simulink model "Naters"  (R2016a)
settings: Solver=FixedStepAuto  StartTime=1  StopTime=60*24*3  FixedStep=1  RelTol=1e-3
InitFcn:
  | %open the initialization function as a structure s
  | model = bdroot;
  | [t,sample_time,k,Text,Text_ini,Tin_sp,rad_90,step,Qdot_dem, Design,T_primary] = system_init(model);
  | %clear ans
  | 
  | 
  | % time vector
  | %t=s.t;
  | t_step = step;
  | time_u = 1;
  | %sample_time = s.sample_time;
  | 
  | % declare parameters
  | Text_D = Design(1);
  | Tin_D = Design(2);
  | Ts_D = Design(3);
  | Tr_D = Design(4);
  | mdot_d_w = Design(5);
  | Qdot_dem = Qdot_dem;
  | %L_ini= L_ini;
  | 
  | %Text_D = s.Design(1);
  | %Tin_D = s.Design(2);
  | %Ts_D = s.Design(3);
  | %Tr_D = s.Design(4);
  | %mdot_d_w = s.Design(5);
  | %Qdot_dem = s.Qdot_dem;
  | %L_ini= s.L_ini;
  | 
  | %Ab_c = Ab_c;
  | %Bb_c = Bb_c;
  | %Tin_sp = Tin_sp.signals.values;
  | Text = Text.signals.values;
  | Rad_90 = rad_90.signals.values;
  | 
  | % k parameters for heat pump model
  | K = k;
values from neighbouring files (symbols this model uses):
  Design = [Text_D, Tin_D, Ts_D, Tr_D, mdot_d_w]    [get_param_building.m]
  k = K    [Frontend.m]    (also in tetsts.m = 2)
  rad_90 = struct('time', t, 'signals', struct('values', rad_90_data(1:length(t))))    [Frontend.m]    (also in system_init.m = kron(rad_90,ones(60,1)); tetsts.m = rad_90(time))
  sample_time = 60    [Frontend.m]    (also in system_init.m = 1; tetsts.m = [1 60 300 900])
  T_primary = 10    [Frontend.m]
undefined symbols (not defined in the file or in its folder): DiscIntNeverNeededParam
libraries: simulink x25, dspsigops x1, carnot x1
(part 1 of 2)
settings Model: Creator=frederic.amblard  LastModifiedBy=frederic.amblard
settings DataIOCC: ExternalInput=[t, Ab_c, Bb_c, Text, Tin_sp]  FinalStateName=NatersV4_cleanV2xFinal  InitialState=NatersV4_cleanV2xFinal  SaveCompleteFinalSimState=on  SaveFormat=Structure

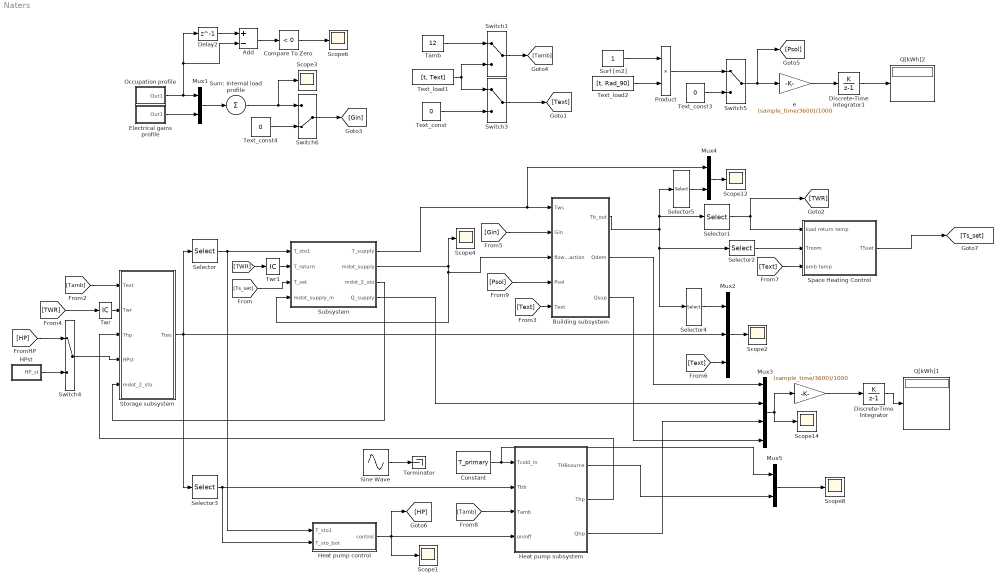
== system Naters ==
  . : Gain  Gain=(sample_time/3600)/1000  SaturateOnIntegerOverflow=on  OutDataTypeStr=Inherit: Same as input  ParamDataTypeStr=Inherit: Same as input
  Add : Sum  Inputs=+-
  Building subsystem : Subsystem
  Compare To Zero : simulink/Logic and Bit Operations/Compare To Zero  relop=<  OutDataTypeStr=uint8
  Constant : Constant  Value=T_primary
  Delay2 : Delay  DelayLength=1  InitialCondition=0
  Discrete-Time Integrator : DiscreteIntegrator  IntegratorMethod=Accumulation: Forward Euler  InitialConditionSetting=State (most efficient)  SampleTime=-1  ICPrevOutput=DiscIntNeverNeededParam  ICPrevScaledInput=DiscIntNeverNeededParam
  Discrete-Time Integrator1 : DiscreteIntegrator  IntegratorMethod=Accumulation: Forward Euler  InitialConditionSetting=State (most efficient)  SampleTime=-1  ICPrevOutput=DiscIntNeverNeededParam  ICPrevScaledInput=DiscIntNeverNeededParam
  Electrical gains profile : Subsystem  mask{period=24*3600/sample_time, rep_seq_t=[0 1 6 7 8 9 11 12 13 18 19 20 22 23]*3600/sample_time, rep_seq_d=[1 5 1 1 1 2 1 1 4 2 1 2 1 1]*3600/sample_time, rep_seq_y=[105 55 392.5 457.5 420 55 250 55 120 170 615 420 442.5 355]*3600/sample_time}
      mask prompts: period "Timeperiod in h"; rep_seq_t "Time values in h"; rep_seq_d "Duration in h"; rep_seq_y "Output values"
  HPst : Subsystem  mask{period=24*3600/sample_time, rep_seq_t=[0 6 7 8 9 11 12 13 14 15 17 18 20 21 22]*3600/sample_time, rep_seq_d=[6 1 1 1 2 1 1 1 1 2 1 2 1 1 2]*3600/sample_time, rep_seq_y=[1 1 1 0 0 0 1 1 1 0 0 1 1 1 1]*3600/sample_time}
      mask prompts: period "Timeperiod in h"; rep_seq_t "Time values in h"; rep_seq_d "Duration in h"; rep_seq_y "Output values"
  Heat pump control : Subsystem
  Heat pump subsystem : Subsystem  mask{K=K, caph=80000, capc=50000, cp=4185, DT=4, UA=7, Qdot_D=Qdot_dem}
      mask prompts: K "Param K"; caph "Thermal capacity hot side [J/K]"; capc "Thermal capacity cold side [J/K]"; cp "Heat capacity of water [J/(kg·K)]"; DT "Delta temperature fixed cold side"; UA "Heat loss coefficient [W/K]"; Qdot_D "Design thermal power [W]"
      mask init:
      | mcdot = 1000*Qdot_D/(DT*cp) / 1000; % mass flow [kg/s]
  Mux1 : Mux  Inputs=2
  Mux2 : Mux  Inputs=3
  Mux3 : Mux
  Mux4 : Mux  Inputs=2
  Mux5 : Mux  Inputs=2
  Occupation profile : Subsystem  mask{period=24*3600/sample_time, rep_seq_t=[0 6 7 8 9 11 12 13 14 15 17 18 20 21 22]*3600/sample_time, rep_seq_d=[6 1 1 1 2 1 1 1 1 2 1 2 1 1 2]*3600/sample_time, rep_seq_y=[4 2 3 2 0 1 3 2 1 0 1 2 4 3 4]*60*3600/sample_time}
      mask prompts: period "Timeperiod in h"; rep_seq_t "Time values in h"; rep_seq_d "Duration in h"; rep_seq_y "Output values"
  Product : Product
  Q[kWh]1 : Display
  Q[kWh]2 : Display
  Scope{1..4,6,8,12,14} (8 alike) : Scope
  Selector : Selector  InputPortWidth=3  IndexOptions=Index vector (dialog)  Indices=[1]  OutputSizes=1
  Selector1 : Selector  InputPortWidth=5  IndexOptions=Index vector (dialog)  Indices=[4]  OutputSizes=1
  Selector2 : Selector  InputPortWidth=5  IndexOptions=Index vector (dialog)  Indices=[5]  OutputSizes=1
  Selector3 : Selector  InputPortWidth=3  IndexOptions=Index vector (dialog)  Indices=[3]  OutputSizes=1
  Selector4 : Selector  InputPortWidth=5  IndexOptions=Index vector (dialog)  Indices=[1, 4, 5]  OutputSizes=1
  Selector5 : Selector  InputPortWidth=5  IndexOptions=Index vector (dialog)  Indices=[1, 2, 3, 4]  OutputSizes=1
  Sine Wave : Sin  SineType=Sample based  Bias=10  Samples=sample_time*100  SampleTime=1  Offset=100
  Space Heating Control : Subsystem  mask{Tset=Tin_D, Tsetn=Tin_D, Q_LOC=Qdot_dem, Td_in=Ts_D, Td_out=Tr_D, Tambd=Text_D, n_rad=1}
      mask prompts: Tset "desired room day Temperature [°C]"; Tsetn "desired room night Temperature [°C]"; Q_LOC "design heat load [W]"; Td_in "design inlet temperature of the heating system [°C]"; Td_out "design outlet temperature of the heating system [°C]"; Tambd "design outdoor temperature"; n_rad "radiatior exponent"
      mask init:
      | dTd = 0.5*(Td_in + Td_out) - Tset;
      | dTdn = 0.5*(Td_in + Td_out) - Tsetn;
  Storage subsystem : Subsystem
  Subsystem : Subsystem
  Sum: Internal load profile : Sum  Inputs=+
  Surf [m2] : Constant
  Switch{1,3..5} (4 alike) : ManualSwitch
  Switch6 : ManualSwitch  CurrentSetting=0
  Tamb : Constant  Value=12
  Terminator : Terminator
  Text_const : Constant  Value=0
  Text_const3 : Constant  Value=0
  Text_const4 : Constant  Value=0
  Text_load1 : FromWorkspace  Tag=Tin_sp  Description=Temperature signal of the room  VariableName=[t, Text]  SampleTime=1  Interpolate=off  OutputAfterFinalValue=Setting to zero
  Text_load2 : FromWorkspace  Tag=Tin_sp  Description=Temperature signal of the room  VariableName=[t, Rad_90]  SampleTime=1  Interpolate=off  OutputAfterFinalValue=Setting to zero
  Twr : InitialCondition  Value=23
  Twr1 : InitialCondition  Value=23
  e : Gain  Gain=(sample_time/3600)/1000  SaturateOnIntegerOverflow=on  OutDataTypeStr=Inherit: Same as input  ParamDataTypeStr=Inherit: Same as input
  wires:
  Text_load1/1 -> Switch1/2, Switch3/1
  Text_const/1 -> Switch3/2
  Switch3/1 -> [Text]
  [Tamb] -> Storage subsystem/1(Text)
  Storage subsystem/1(Ttes) -> Selector3/1, Mux2/2, Selector/1
  Occupation profile/1(Out1) -> Add/2, Delay2/1, Mux1/1
  Electrical gains profile/1(Out1) -> Mux1/2
  Mux1/1 -> Sum: Internal load profile/1
  Sum: Internal load profile/1 -> Scope3/1, Switch6/1
  Building subsystem/1(Tb_out) -> Selector2/1, Selector4/1, Selector5/1, Selector1/1
  Selector1/1 -> [TWR], Space Heating Control/1(load return temp)
  [TWR] -> Twr/1
  Twr/1 -> Storage subsystem/2(Twr)
  [Gin] -> Building subsystem/2(Gin)
  Text_load2/1 -> Product/2
  Mux2/1 -> Scope2/1
  HPst/1(HP_st) -> Switch4/2
  [Text] -> Mux2/3
  Tamb/1 -> Switch1/1
  Switch1/1 -> [Tamb]
  Selector2/1 -> Space Heating Control/2(Troom)
  [Text] -> Space Heating Control/3(amb temp)
  ? -> ?
  Switch4/1 -> Storage subsystem/4(HPst)
  [HP] -> Switch4/1
  Selector3/1 -> Heat pump subsystem/2(Tbb), Heat pump control/2(T_sto_bot)
  [Tamb] -> Heat pump subsystem/3(Tamb)
  Heat pump control/1(control) -> [HP], Scope1/1, Heat pump subsystem/4(on/off)
  Heat pump subsystem/1(THBsource) -> Mux5/2
  Heat pump subsystem/2(Thp) -> Storage subsystem/3(Thp)
  Sine Wave/1 -> Terminator/1
  Surf [m2]/1 -> Product/1
  Product/1 -> Switch5/1
  [Psol] -> Building subsystem/4(Psol)
  Building subsystem/2(Qdem) -> Mux3/1
  Selector/1 -> Subsystem/1(T_sto1), Heat pump control/1(T_sto1)
  Mux3/1 -> ./1, Scope14/1
  Discrete-Time Integrator/1 -> Q[kWh]1/1
  ./1 -> Discrete-Time Integrator/1
  Text_const3/1 -> Switch5/2
  Switch5/1 -> [Psol], e/1
  Text_const4/1 -> Switch6/2
  Switch6/1 -> [Gin]
  Heat pump subsystem/3(Qhp) -> Mux3/3
  [Text] -> Building subsystem/5(Text)
  Delay2/1 -> Add/1
  Add/1 -> Compare To Zero/1
  Compare To Zero/1 -> Scope6/1
  [TWR] -> Twr1/1
  [Ts_set] -> Subsystem/3(T_set)
  Subsystem/3(mdot_2_sto) -> Storage subsystem/5(mdot_2_sto)
  Subsystem/2(mdot_supply) -> Subsystem/4(mdot_supply_in), Building subsystem/3(flow_fraction), Scope4/1
  Subsystem/4(Q_supply) -> Mux3/2
  Twr1/1 -> Subsystem/2(T_return)
  Subsystem/1(T_supply) -> Mux4/1, Building subsystem/1(Tws)
  Selector4/1 -> Mux2/1
  Selector5/1 -> Mux4/2
  Mux4/1 -> Scope12/1
  Space Heating Control/1(TSset) -> [Ts_set]
  e/1 -> Discrete-Time Integrator1/1
  Discrete-Time Integrator1/1 -> Q[kWh]2/1
  Building subsystem/3(Qsup) -> Mux3/4
  Mux5/1 -> Scope8/1
  Constant/1 -> Mux5/1, Heat pump subsystem/1(Tcold_in)

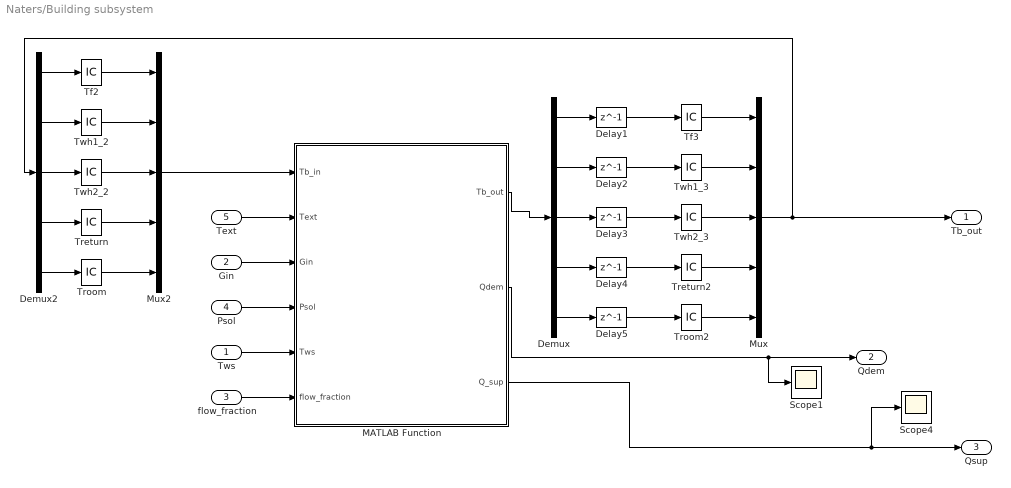
== system Naters/Building subsystem ==
  Tws : Inport
  Gin : Inport  Port=2
  flow_fraction : Inport  Port=3
  Psol : Inport  Port=4
  Text : Inport  Port=5
  Delay1 : Delay  DelayLength=1  InitialCondition=0  InputProcessing=Inherited
  Delay2 : Delay  DelayLength=1  InitialCondition=0  InputProcessing=Inherited
  Delay3 : Delay  DelayLength=1  InitialCondition=0
  Delay4 : Delay  DelayLength=1  InitialCondition=0  InputProcessing=Inherited
  Delay5 : Delay  DelayLength=1  InitialCondition=0
  Demux : Demux  Outputs=5
  Demux2 : Demux  Outputs=5
  MATLAB Function : MATLAB Function  TreatAsAtomicUnit=on  mask{sample_time=sample_time}
  Mux : Mux  Inputs=5
  Mux2 : Mux  Inputs=5
  Scope1 : Scope
  Scope4 : Scope
  Tf2 : InitialCondition  Value=22
  Tf3 : InitialCondition  Value=22
  Treturn : InitialCondition  Value=23
  Treturn2 : InitialCondition  Value=23
  Troom : InitialCondition  Value=20
  Troom2 : InitialCondition  Value=20
  Twh1_2 : InitialCondition  Value=25
  Twh1_3 : InitialCondition  Value=25
  Twh2_2 : InitialCondition  Value=24
  Twh2_3 : InitialCondition  Value=24
  Tb_out : Outport
  Qdem : Outport  Port=2
  Qsup : Outport  Port=3
  wires:
  MATLAB Function/1(Tb_out) -> Demux/1
  Demux/2 -> Delay2/1
  Demux/3 -> Delay3/1
  flow_fraction/1 -> MATLAB Function/6(flow_fraction)
  Gin/1 -> MATLAB Function/3(Gin)
  Psol/1 -> MATLAB Function/4(Psol)
  MATLAB Function/2(Qdem) -> Scope1/1, Qdem/1
  Tws/1 -> MATLAB Function/5(Tws)
  Text/1 -> MATLAB Function/2(Text)
  Demux/1 -> Delay1/1
  Demux2/2 -> Twh1_2/1
  Demux2/3 -> Twh2_2/1
  Mux2/1 -> MATLAB Function/1(Tb_in)
  Twh1_2/1 -> Mux2/2
  Twh2_2/1 -> Mux2/3
  Demux2/1 -> Tf2/1
  Tf2/1 -> Mux2/1
  Demux2/4 -> Treturn/1
  Demux2/5 -> Troom/1
  Demux/4 -> Delay4/1
  Demux/5 -> Delay5/1
  Treturn/1 -> Mux2/4
  Troom/1 -> Mux2/5
  Mux/1 -> Demux2/1, Tb_out/1
  Delay2/1 -> Twh1_3/1
  Delay3/1 -> Twh2_3/1
  Delay1/1 -> Tf3/1
  Delay4/1 -> Treturn2/1
  Delay5/1 -> Troom2/1
  Treturn2/1 -> Mux/4
  Twh1_3/1 -> Mux/2
  Troom2/1 -> Mux/5
  Tf3/1 -> Mux/1
  Twh2_3/1 -> Mux/3
  MATLAB Function/3(Q_sup) -> Scope4/1, Qsup/1

== system Naters/Electrical gains profile ==
  Pulse Generator : DiscretePulseGenerator  PulseType=Time based  Amplitude=rep_seq_y  Period=period  PulseWidth=rep_seq_d*100/period  PhaseDelay=rep_seq_t
  Sum of Elements : Sum  Inputs=+
  Out1 : Outport
  wires:
  Sum of Elements/1 -> Out1/1
  Pulse Generator/1 -> Sum of Elements/1

== system Naters/HPst ==
  Pulse Generator : DiscretePulseGenerator  PulseType=Time based  Amplitude=rep_seq_y  Period=period  PulseWidth=rep_seq_d*100/period  PhaseDelay=rep_seq_t
  Sum of Elements : Sum  Inputs=+
  HP_st : Outport
  wires:
  Sum of Elements/1 -> HP_st/1
  Pulse Generator/1 -> Sum of Elements/1

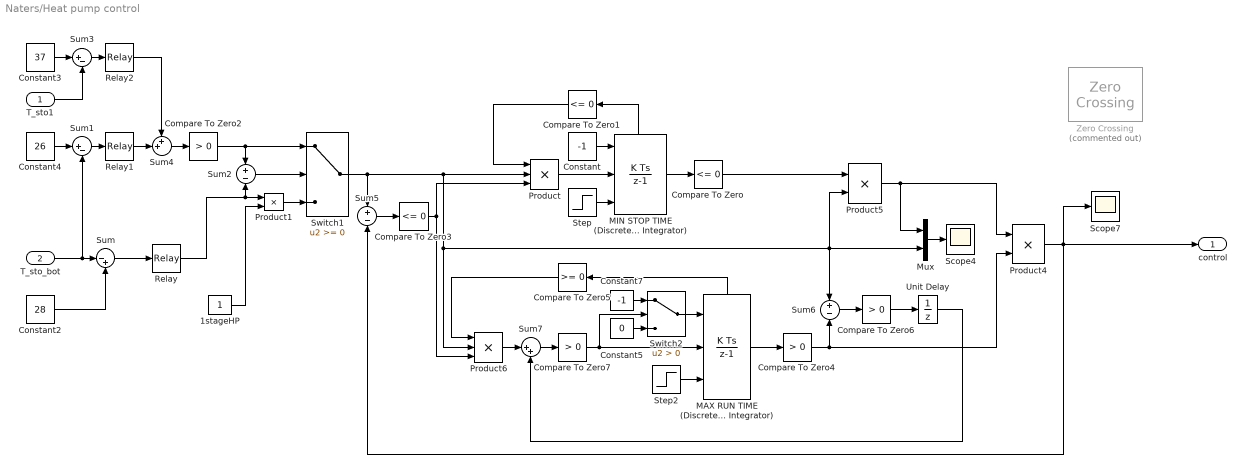
== system Naters/Heat pump control ==
  T_sto1 : Inport
  T_sto_bot : Inport  Port=2
  1stageHP : Constant
  Compare To Zero : simulink/Logic and Bit Operations/Compare To Zero  relop=<=  OutDataTypeStr=uint8
  Compare To Zero1 : simulink/Logic and Bit Operations/Compare To Zero  relop=<=  OutDataTypeStr=uint8
  Compare To Zero2 : simulink/Logic and Bit Operations/Compare To Zero  relop=>  OutDataTypeStr=boolean
  Compare To Zero3 : simulink/Logic and Bit Operations/Compare To Zero  relop=<=  OutDataTypeStr=uint8
  Compare To Zero4 : simulink/Logic and Bit Operations/Compare To Zero  relop=>  OutDataTypeStr=uint8
  Compare To Zero5 : simulink/Logic and Bit Operations/Compare To Zero  relop=>=  OutDataTypeStr=uint8
  Compare To Zero6 : simulink/Logic and Bit Operations/Compare To Zero  relop=>  OutDataTypeStr=uint8
  Compare To Zero7 : simulink/Logic and Bit Operations/Compare To Zero  relop=>  OutDataTypeStr=uint8
  Constant : Constant  Value=-1
  Constant2 : Constant  Value=28
  Constant3 : Constant  Value=37
  Constant4 : Constant  Value=26
  Constant5 : Constant  Value=0  SampleTime=-1
  Constant7 : Constant  Value=-1  SampleTime=-1
  MAX RUN TIME (Discrete-Time Integrator) : DiscreteIntegrator  ExternalReset=falling  InitialConditionSource=external  InitialConditionSetting=State (most efficient)  SampleTime=-1  LowerSaturationLimit=0  ShowStatePort=on  IgnoreLimit=on  ICPrevOutput=DiscIntNeverNeededParam  ICPrevScaledInput=DiscIntNeverNeededParam
  MIN STOP TIME (Discrete-Time Integrator) : DiscreteIntegrator  ExternalReset=falling  InitialConditionSource=external  InitialConditionSetting=State (most efficient)  SampleTime=-1  LimitOutput=on  LowerSaturationLimit=0  ShowStatePort=on  ICPrevOutput=DiscIntNeverNeededParam  ICPrevScaledInput=DiscIntNeverNeededParam
  Mux : Mux  Inputs=2
  Product : Product  Inputs=3  RndMeth=Zero
  Product1 : Product  RndMeth=Zero
  Product4 : Product  RndMeth=Zero
  Product5 : Product  RndMeth=Zero
  Product6 : Product  Inputs=3  RndMeth=Zero
  Relay : Relay  OnSwitchValue=1  OffSwitchValue=-6
  Relay1 : Relay  OnSwitchValue=1  OffSwitchValue=-2
  Relay2 : Relay  OnSwitchValue=1  OffSwitchValue=-6
  Scope4 : Scope
  Scope7 : Scope
  Step : Step  After=(15*60)/sample_time  SampleTime=1
  Step2 : Step  After=180000/sample_time  SampleTime=1  VectorParams1D=off
  Sum : Sum  Inputs=|-+
  Sum1 : Sum  Inputs=|+-
  Sum2 : Sum  Inputs=+|-
  Sum3 : Sum  Inputs=|+-
  Sum4 : Sum  Inputs=++|
  Sum5 : Sum  Inputs=+|-
  Sum6 : Sum  Inputs=+|-
  Sum7 : Sum  Inputs=|++
  Switch1 : Switch
  Switch2 : Switch  Criteria=u2 > Threshold
  Unit Delay : UnitDelay  SampleTime=-1
  Zero Crossing : dspsigops/Zero Crossing  Commented=on  InputProcessing=Columns as channels (frame based)
  control : Outport
  wires:
  T_sto_bot/1 -> Sum/1, Sum1/2
  Constant2/1 -> Sum/2
  Sum/1 -> Relay/1
  Product/1 -> MIN STOP TIME (Discrete-Time Integrator)/2
  MIN STOP TIME (Discrete-Time Integrator)/State -> Compare To Zero1/1
  Constant/1 -> MIN STOP TIME (Discrete-Time Integrator)/1
  Step/1 -> MIN STOP TIME (Discrete-Time Integrator)/3
  MIN STOP TIME (Discrete-Time Integrator)/1 -> Compare To Zero/1
  Mux/1 -> Scope4/1
  Compare To Zero/1 -> Product5/1
  Product5/1 -> Mux/1, Product4/1
  MAX RUN TIME (Discrete-Time Integrator)/State -> Compare To Zero5/1
  Step2/1 -> MAX RUN TIME (Discrete-Time Integrator)/3
  Relay/1 -> Product1/1, Sum2/2
  1stageHP/1 -> Product1/2
  Constant4/1 -> Sum1/1
  Sum1/1 -> Relay1/1
  Sum4/1 -> Compare To Zero2/1
  Product1/1 -> Switch1/3
  Sum2/1 -> Switch1/2
  Constant3/1 -> Sum3/1
  T_sto1/1 -> Sum3/2
  Sum3/1 -> Relay2/1
  Relay2/1 -> Sum4/1
  Relay1/1 -> Sum4/2
  Compare To Zero2/1 -> Switch1/1, Sum2/1
  Switch1/1 -> Product/2, Product6/2, Product5/2, Mux/2, Sum6/1, Sum5/1
  Sum5/1 -> Compare To Zero3/1
  Sum6/1 -> Compare To Zero6/1
  Product6/1 -> Sum7/1
  Compare To Zero6/1 -> Unit Delay/1
  Compare To Zero4/1 -> Sum6/2, Product4/2
  Compare To Zero3/1 -> Product/3, Product6/3
  Sum7/1 -> Compare To Zero7/1
  Compare To Zero7/1 -> Switch2/2, MAX RUN TIME (Discrete-Time Integrator)/2
  Unit Delay/1 -> Sum7/2
  Constant7/1 -> Switch2/1
  Compare To Zero5/1 -> Product6/1
  MAX RUN TIME (Discrete-Time Integrator)/1 -> Compare To Zero4/1
  Switch2/1 -> MAX RUN TIME (Discrete-Time Integrator)/1
  Constant5/1 -> Switch2/3
  Compare To Zero1/1 -> Product/1
  Product4/1 -> Sum5/2, control/1, Scope7/1

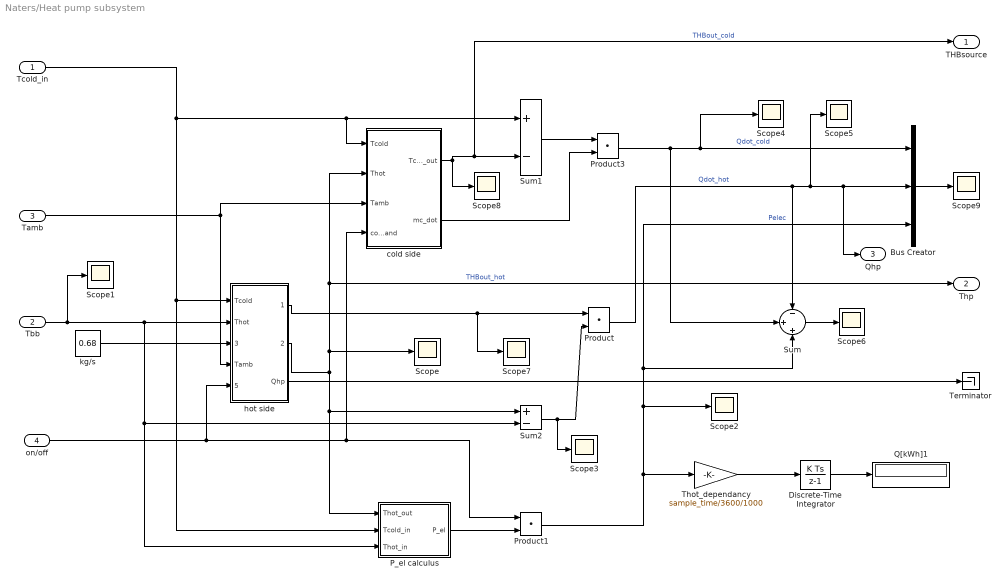
== system Naters/Heat pump subsystem ==
  Tcold_in : Inport
  Tbb : Inport  Port=2
  Tamb : Inport  Port=3
  on/off : Inport  Port=4
  Bus Creator : BusCreator  Inputs=3
  Discrete-Time Integrator : DiscreteIntegrator  InitialConditionSetting=State (most efficient)  SampleTime=-1  ICPrevOutput=DiscIntNeverNeededParam  ICPrevScaledInput=DiscIntNeverNeededParam
  P_el calculus : Subsystem  AncestorBlock=carnot/Basic/Thermal_Models/HeatPump_basic/P_el calculus
  Product : DotProduct  InputSameDT=on  OutDataTypeStr=Inherit: Inherit via internal rule
  Product1 : DotProduct  InputSameDT=on  OutDataTypeStr=Inherit: Inherit via internal rule
  Product3 : DotProduct  InputSameDT=on  OutDataTypeStr=Inherit: Inherit via internal rule
  Q[kWh]1 : Display
  Scope{,1..9} (10 alike) : Scope
  Sum : Sum  Inputs=-|+|+
  Sum1 : Sum  Inputs=+-  SaturateOnIntegerOverflow=on  InputSameDT=on  OutDataTypeStr=Inherit: Same as first input
  Sum2 : Sum  Inputs=+-  SaturateOnIntegerOverflow=on  InputSameDT=on  OutDataTypeStr=Inherit: Same as first input
  Terminator : Terminator
  Thot_dependancy : Gain  Gain=sample_time/3600/1000  SaturateOnIntegerOverflow=on  OutDataTypeStr=Inherit: Same as input  ParamDataTypeStr=Inherit: Same as input
  cold side : Subsystem
  hot side : Subsystem
  kg/s : Constant  Value=0.68
  THBsource : Outport
  Thp : Outport  Port=2
  Qhp : Outport  Port=3
  wires:
  Bus Creator/1 -> Scope9/1
  cold side/1(Tcold_out) -> THBsource/1, Sum1/2, Scope8/1  "THBout_cold"
  hot side/2(Thot_out) -> cold side/2(Thot), Thp/1, Scope/1, P_el calculus/1(Thot_out), Sum2/1  "THBout_hot"
  Tamb/1 -> cold side/3(Tamb), hot side/4(Tamb)
  Tbb/1 -> Scope1/1, hot side/2(Thot), P_el calculus/3(Thot_in), Sum2/2
  hot side/1(mdot*cp) -> Scope7/1, Product/1
  Sum2/1 -> Scope3/1, Product/2
  Tcold_in/1 -> hot side/1(Tcold), P_el calculus/2(Tcold_in), cold side/1(Tcold), Sum1/1
  P_el calculus/1(P_el) -> Product1/2
  Product1/1 -> Thot_dependancy/1, Scope2/1, Sum/3, Bus Creator/3  "Pelec"
  on/off/1 -> hot side/5(command), cold side/4(command), Product1/1
  Sum1/1 -> Product3/1
  Product3/1 -> Sum/2, Scope4/1, Bus Creator/1  "Qdot_cold"
  Product/1 -> Sum/1, Scope5/1, Qhp/1, Bus Creator/2  "Qdot_hot"
  kg/s/1 -> hot side/3(mdot_hot)
  Discrete-Time Integrator/1 -> Q[kWh]1/1
  Thot_dependancy/1 -> Discrete-Time Integrator/1
  Sum/1 -> Scope6/1
  hot side/3(Qhp) -> Terminator/1
  cold side/2(mc_dot) -> Product3/2

== system Naters/Occupation profile ==
  Pulse Generator : DiscretePulseGenerator  PulseType=Time based  Amplitude=rep_seq_y  Period=period  PulseWidth=rep_seq_d*100/period  PhaseDelay=[0 6 7 8 9 11 12 13 14 15 17 18 20 21 22]*3600/sample_time  VectorParams1D=off
  Pulse Generator1 : DiscretePulseGenerator  Commented=on  Amplitude=[4000 7000]  Period=60*24/sample_time  PulseWidth="[100 20 ;  200]"  PhaseDelay=[100 200]  VectorParams1D=off
  Pulse Generator2 : DiscretePulseGenerator  Commented=on  PulseType=Time based  Amplitude=rep_seq_y  Period=24*60/sample_time  PulseWidth=|  PhaseDelay=[0 6 7 8 9 11 12 13 14 15 17 18 20 21 22]*60/sample_time  VectorParams1D=off
      | [25.00000 4.16666 4.16666 4.16666 8.33333 4.16666 4.16666 4.16666 4.16666 8.33333 4.16666 8.33333
      | 4.16666 4.16666 8.33333]
  Scope1 : Scope
  Scope{2..3,5..6} (4 alike) : Scope  Commented=on
  Scope4 : Scope
  Sum of Elements : Sum  Inputs=+  RndMeth=Round
  Sum of Elements1 : Sum  Commented=on  Inputs=+  RndMeth=Round
  Sum of Elements2 : Sum  Commented=on  Inputs=+  RndMeth=Round
  Out1 : Outport
  wires:
  Sum of Elements/1 -> Scope1/1, Out1/1
  Pulse Generator/1 -> Scope4/1, Sum of Elements/1
  Sum of Elements1/1 -> Scope2/1
  Pulse Generator1/1 -> Scope3/1, Sum of Elements1/1
  Sum of Elements2/1 -> Scope5/1
  Pulse Generator2/1 -> Scope6/1, Sum of Elements2/1

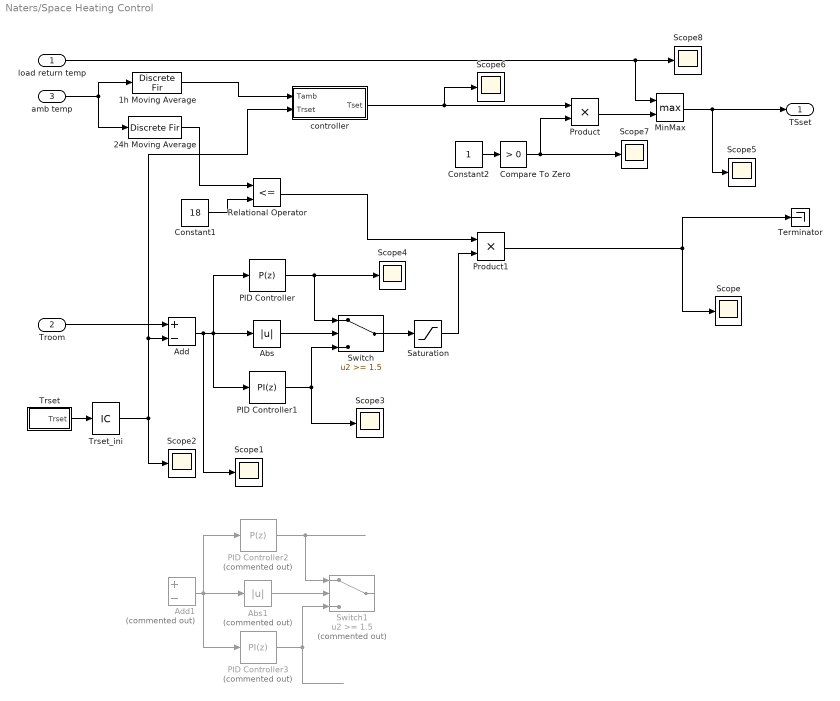
== system Naters/Space Heating Control ==
  load return temp : Inport
  Troom : Inport  Port=2
  amb temp : Inport  Port=3
  1h Moving Average : DiscreteFir  Coefficients=ones(1,3600/sample_time*1)*(1/((3600/sample_time)*1))  SampleTime=1  AccumDataTypeStr=Inherit: Same as product output  RndMeth=Nearest
  24h Moving Average : DiscreteFir  Coefficients=ones(1,3600/sample_time*24)*(1/((3600/sample_time)*24))  SampleTime=1  AccumDataTypeStr=Inherit: Same as product output  RndMeth=Nearest
  Abs : Abs
  Abs1 : Abs  Commented=on
  Add : Sum  Inputs=+-
  Add1 : Sum  Commented=on  Inputs=+-
  Compare To Zero : simulink/Logic and Bit Operations/Compare To Zero  relop=>  OutDataTypeStr=boolean
  Constant1 : Constant  Value=18
  Constant2 : Constant
  MinMax : MinMax  Function=max  Inputs=2
  PID Controller : simulink/Continuous/PID Controller  Controller=P  TimeDomain=Discrete-time  SampleTime=-1  IntegratorMethod=Forward Euler  FilterMethod=Forward Euler  Form=Parallel  UseFilter=on  ControllerParametersSource=internal  P=-0.6  I=1  D=0  N=100  InitialConditionSource=internal  InitialConditionForIntegrator=0  InitialConditionForFilter=0  ExternalReset=none  ZeroCross=off  LimitOutput=on  UpperSaturationLimit=1  LowerSaturationLimit=0  LinearizeAsGain=off  AntiWindupMode=none  Kb=1  TrackingMode=off  Kt=1  PParamMin=[]  PParamMax=[]  IParamMin=[]  IParamMax=[]  DParamMin=[]  DParamMax=[]  NParamMin=[]  NParamMax=[]  KbParamMin=[]  KbParamMax=[]  KtParamMin=[]  KtParamMax=[]  POutMin=[]  POutMax=[]  IOutMin=[]  IOutMax=[]  DOutMin=[]  DOutMax=[]  NOutMin=[]  NOutMax=[]  KbOutMin=[]  KbOutMax=[]  KtOutMin=[]  KtOutMax=[]  IntegratorOutMin=[]  IntegratorOutMax=[]  FilterOutMin=[]  FilterOutMax=[]  SumOutMin=[]  SumOutMax=[]  SumI1OutMin=[]  SumI1OutMax=[]  SumI2OutMin=[]  SumI2OutMax=[]  SumI3OutMin=[]  SumI3OutMax=[]  SumDOutMin=[]  SumDOutMax=[]  SaturationOutMin=[]  SaturationOutMax=[]  IntegratorContinuousStateAttributes=''  IntegratorStateMustResolveToSignalObject=off  IntegratorRTWStateStorageClass=Auto  FilterContinuousStateAttributes=''  FilterStateMustResolveToSignalObject=off  FilterRTWStateStorageClass=Auto  DifferentiatorICPrevScaledInput=0  DifferentiatorOutMin=[]  DifferentiatorOutMax=[]
  PID Controller1 : simulink/Continuous/PID Controller  Controller=PI  TimeDomain=Discrete-time  SampleTime=-1  IntegratorMethod=Backward Euler  FilterMethod=Forward Euler  Form=Parallel  UseFilter=on  ControllerParametersSource=internal  P=-0.9  I=-0.2/(3600/(sample_time))  D=0.001  N=100  InitialConditionSource=internal  InitialConditionForIntegrator=0  InitialConditionForFilter=0  ExternalReset=none  LimitOutput=on  UpperSaturationLimit=1  LowerSaturationLimit=0  LinearizeAsGain=off  AntiWindupMode=back-calculation  Kb=1  TrackingMode=off  Kt=1  PParamMin=[]  PParamMax=[]  IParamMin=[]  IParamMax=[]  DParamMin=[]  DParamMax=[]  NParamMin=[]  NParamMax=[]  KbParamMin=[]  KbParamMax=[]  KtParamMin=[]  KtParamMax=[]  POutMin=[]  POutMax=[]  IOutMin=[]  IOutMax=[]  DOutMin=[]  DOutMax=[]  NOutMin=[]  NOutMax=[]  KbOutMin=[]  KbOutMax=[]  KtOutMin=[]  KtOutMax=[]  IntegratorOutMin=[]  IntegratorOutMax=[]  FilterOutMin=[]  FilterOutMax=[]  SumOutMin=[]  SumOutMax=[]  SumI1OutMin=[]  SumI1OutMax=[]  SumI2OutMin=[]  SumI2OutMax=[]  SumI3OutMin=[]  SumI3OutMax=[]  SumDOutMin=[]  SumDOutMax=[]  SaturationOutMin=[]  SaturationOutMax=[]  IntegratorContinuousStateAttributes=''  IntegratorStateMustResolveToSignalObject=off  IntegratorRTWStateStorageClass=Auto  FilterContinuousStateAttributes=''  FilterStateMustResolveToSignalObject=off  FilterRTWStateStorageClass=Auto  DifferentiatorICPrevScaledInput=0  DifferentiatorOutMin=[]  DifferentiatorOutMax=[]
  PID Controller2 : simulink/Continuous/PID Controller  Commented=on  Controller=P  TimeDomain=Discrete-time  SampleTime=-1  IntegratorMethod=Forward Euler  FilterMethod=Forward Euler  Form=Parallel  UseFilter=on  ControllerParametersSource=internal  P=-0.5  I=1  D=0  N=100  InitialConditionSource=internal  InitialConditionForIntegrator=0  InitialConditionForFilter=0  ExternalReset=none  ZeroCross=off  LimitOutput=on  UpperSaturationLimit=1  LowerSaturationLimit=0  LinearizeAsGain=off  AntiWindupMode=none  Kb=1  TrackingMode=off  Kt=1  PParamMin=[]  PParamMax=[]  IParamMin=[]  IParamMax=[]  DParamMin=[]  DParamMax=[]  NParamMin=[]  NParamMax=[]  KbParamMin=[]  KbParamMax=[]  KtParamMin=[]  KtParamMax=[]  POutMin=[]  POutMax=[]  IOutMin=[]  IOutMax=[]  DOutMin=[]  DOutMax=[]  NOutMin=[]  NOutMax=[]  KbOutMin=[]  KbOutMax=[]  KtOutMin=[]  KtOutMax=[]  IntegratorOutMin=[]  IntegratorOutMax=[]  FilterOutMin=[]  FilterOutMax=[]  SumOutMin=[]  SumOutMax=[]  SumI1OutMin=[]  SumI1OutMax=[]  SumI2OutMin=[]  SumI2OutMax=[]  SumI3OutMin=[]  SumI3OutMax=[]  SumDOutMin=[]  SumDOutMax=[]  SaturationOutMin=[]  SaturationOutMax=[]  IntegratorContinuousStateAttributes=''  IntegratorStateMustResolveToSignalObject=off  IntegratorRTWStateStorageClass=Auto  FilterContinuousStateAttributes=''  FilterStateMustResolveToSignalObject=off  FilterRTWStateStorageClass=Auto  DifferentiatorICPrevScaledInput=0  DifferentiatorOutMin=[]  DifferentiatorOutMax=[]
  PID Controller3 : simulink/Continuous/PID Controller  Commented=on  Controller=PI  TimeDomain=Discrete-time  SampleTime=-1  IntegratorMethod=Backward Euler  FilterMethod=Forward Euler  Form=Parallel  UseFilter=on  ControllerParametersSource=internal  P=-0.6  I=-0.05/(60*sample_time)  D=0.001  N=100  InitialConditionSource=internal  InitialConditionForIntegrator=0  InitialConditionForFilter=0  ExternalReset=none  ZeroCross=off  LimitOutput=on  UpperSaturationLimit=1  LowerSaturationLimit=0  LinearizeAsGain=off  AntiWindupMode=back-calculation  Kb=1  TrackingMode=off  Kt=1  PParamMin=[]  PParamMax=[]  IParamMin=[]  IParamMax=[]  DParamMin=[]  DParamMax=[]  NParamMin=[]  NParamMax=[]  KbParamMin=[]  KbParamMax=[]  KtParamMin=[]  KtParamMax=[]  POutMin=[]  POutMax=[]  IOutMin=[]  IOutMax=[]  DOutMin=[]  DOutMax=[]  NOutMin=[]  NOutMax=[]  KbOutMin=[]  KbOutMax=[]  KtOutMin=[]  KtOutMax=[]  IntegratorOutMin=[]  IntegratorOutMax=[]  FilterOutMin=[]  FilterOutMax=[]  SumOutMin=[]  SumOutMax=[]  SumI1OutMin=[]  SumI1OutMax=[]  SumI2OutMin=[]  SumI2OutMax=[]  SumI3OutMin=[]  SumI3OutMax=[]  SumDOutMin=[]  SumDOutMax=[]  SaturationOutMin=[]  SaturationOutMax=[]  IntegratorContinuousStateAttributes=''  IntegratorStateMustResolveToSignalObject=off  IntegratorRTWStateStorageClass=Auto  FilterContinuousStateAttributes=''  FilterStateMustResolveToSignalObject=off  FilterRTWStateStorageClass=Auto  DifferentiatorICPrevScaledInput=0  DifferentiatorOutMin=[]  DifferentiatorOutMax=[]
  Product : Product
  Product1 : Product
  Relational Operator : RelationalOperator  Operator=<=  OutDataTypeStr=boolean
  Saturation : Saturate  UpperLimit=1  LowerLimit=0  LinearizeAsGain=off  ZeroCross=off
  Scope{,1..8} (9 alike) : Scope
  Switch : Switch  Threshold=1.5
  Switch1 : Switch  Commented=on  Threshold=1.5
  Terminator : Terminator
  Trset : Subsystem  mask{period=24*3600/sample_time, rep_seq_t=[0 7 21]*3600/sample_time, rep_seq_d=[7 14 3]*3600/sample_time, rep_seq_y=[Tsetn Tset Tsetn]}
      mask prompts: period "Timeperiod in h"; rep_seq_t "Time values in h"; rep_seq_d "Duration in h"; rep_seq_y "Output values"
  Trset_ini : InitialCondition  Value=19.9
  controller : Subsystem
  TSset : Outport
  wires:
  amb temp/1 -> 24h Moving Average/1, 1h Moving Average/1
  Constant1/1 -> Relational Operator/2
  Troom/1 -> Add/1
  Add/1 -> Scope1/1, PID Controller/1, PID Controller1/1, Abs/1
  Abs/1 -> Switch/2
  PID Controller/1 -> Scope4/1, Switch/1
  PID Controller1/1 -> Switch/3, Scope3/1
  Switch/1 -> Saturation/1
  Saturation/1 -> Product1/2
  Product/1 -> MinMax/2
  load return temp/1 -> Scope8/1, MinMax/1
  Compare To Zero/1 -> Product/2, Scope7/1
  24h Moving Average/1 -> Relational Operator/1
  controller/1(Tset) -> Scope6/1, Product/1
  Relational Operator/1 -> Product1/1
  Trset/1(Trset) -> Trset_ini/1
  Add1/1 -> PID Controller2/1, PID Controller3/1, Abs1/1
  Abs1/1 -> Switch1/2
  PID Controller2/1 -> Switch1/1
  PID Controller3/1 -> Switch1/3
  Trset_ini/1 -> controller/2(Trset), Add/2, Scope2/1
  Product1/1 -> Terminator/1, Scope/1
  MinMax/1 -> TSset/1, Scope5/1
  1h Moving Average/1 -> controller/1(Tamb)
  Constant2/1 -> Compare To Zero/1

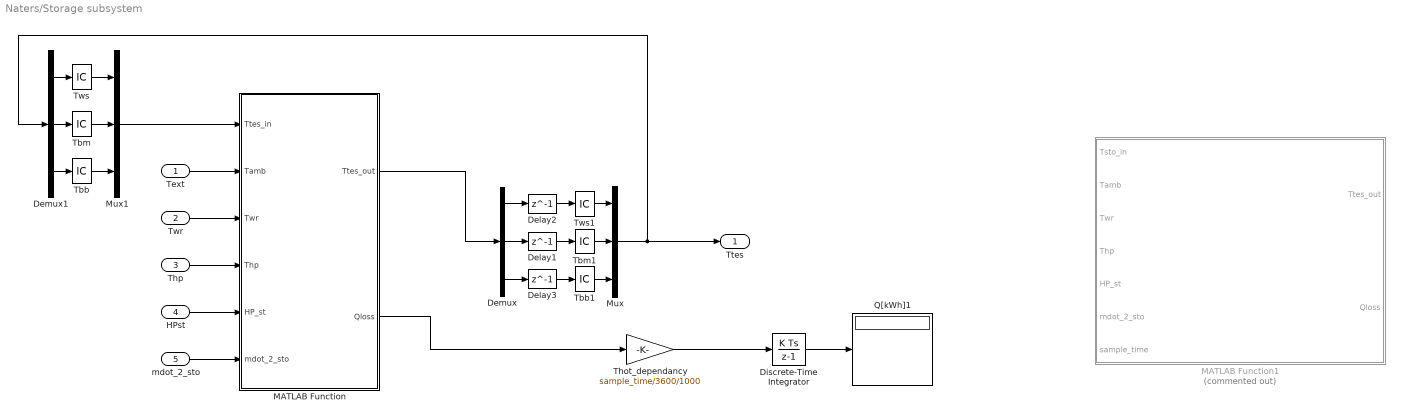
== system Naters/Storage subsystem ==
  Text : Inport
  Twr : Inport  Port=2
  Thp : Inport  Port=3
  HPst : Inport  Port=4
  mdot_2_sto : Inport  Port=5
  Delay1 : Delay  DelayLength=1  InitialCondition=0
  Delay2 : Delay  DelayLength=1  InitialCondition=0
  Delay3 : Delay  DelayLength=1  InitialCondition=0
  Demux : Demux  Outputs=3
  Demux1 : Demux  Outputs=3
  Discrete-Time Integrator : DiscreteIntegrator  InitialConditionSetting=State (most efficient)  SampleTime=-1  ICPrevOutput=DiscIntNeverNeededParam  ICPrevScaledInput=DiscIntNeverNeededParam
  MATLAB Function : MATLAB Function  TreatAsAtomicUnit=on  mask{sample_time=sample_time}
      mask prompts: sample_time "sampling_time"
  MATLAB Function1 : MATLAB Function  Commented=on  TreatAsAtomicUnit=on  mask{sample_time=sample_time, h_sto=2, V_sto=1.2, nb_nodes=6, nb_loops=2, loop_in_out=[ 1 6 ; 6 1 ]}
      mask prompts: sample_time "sampling_time"; h_sto "Height [m]"; V_sto "Volume [m3]"; nb_nodes "Nb Nodes"; nb_loops "Nb Loops"; loop_in_out "Loop geometry [in1 out1;in2 out2]"
  Mux : Mux  Inputs=3
  Mux1 : Mux  Inputs=3
  Q[kWh]1 : Display
  Tbb : InitialCondition  Value=28
  Tbb1 : InitialCondition  Value=28
  Tbm : InitialCondition  Value=31
  Tbm1 : InitialCondition  Value=31
  Thot_dependancy : Gain  Gain=sample_time/3600/1000  SaturateOnIntegerOverflow=on  OutDataTypeStr=Inherit: Same as input  ParamDataTypeStr=Inherit: Same as input
  Tws : InitialCondition  Value=35
  Tws1 : InitialCondition  Value=35
  Ttes : Outport
  wires:
  MATLAB Function/1(Ttes_out) -> Demux/1
  Delay2/1 -> Tws1/1
  Delay1/1 -> Tbm1/1
  Text/1 -> MATLAB Function/2(Tamb)
  HPst/1 -> MATLAB Function/5(HP_st)
  mdot_2_sto/1 -> MATLAB Function/6(mdot_2_sto)
  Demux/1 -> Delay2/1
  Demux/2 -> Delay1/1
  Demux1/2 -> Tbm/1
  Tbm/1 -> Mux1/2
  Demux1/1 -> Tws/1
  Tws/1 -> Mux1/1
  Mux1/1 -> MATLAB Function/1(Ttes_in)
  Thp/1 -> MATLAB Function/4(Thp)
  Twr/1 -> MATLAB Function/3(Twr)
  Discrete-Time Integrator/1 -> Q[kWh]1/1
  Thot_dependancy/1 -> Discrete-Time Integrator/1
  MATLAB Function/2(Qloss) -> Thot_dependancy/1
  Demux/3 -> Delay3/1
  Delay3/1 -> Tbb1/1
  Demux1/3 -> Tbb/1
  Tbb/1 -> Mux1/3
  Mux/1 -> Ttes/1, Demux1/1
  Tws1/1 -> Mux/1
  Tbm1/1 -> Mux/2
  Tbb1/1 -> Mux/3

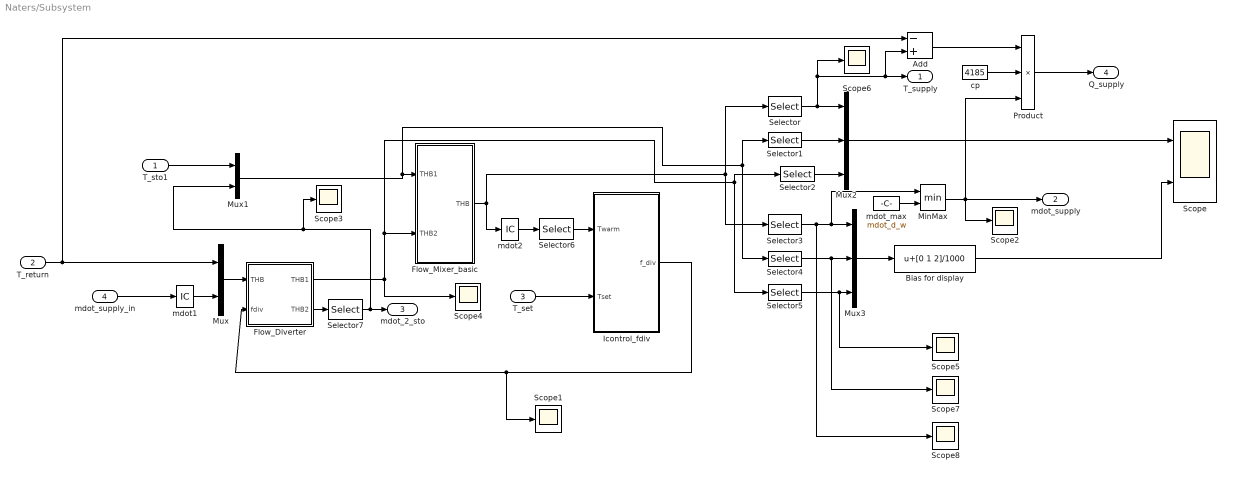
== system Naters/Subsystem ==
  T_sto1 : Inport
  T_return : Inport  Port=2
  T_set : Inport  Port=3
  mdot_supply_in : Inport  Port=4
  Add : Sum  Inputs=-+
  Bias for display : Bias  Bias=[0 1 2]/1000
  Flow_Diverter : Subsystem  mask(flow diverter, fixed rate){}
      mask help:
      | The block diverts an incoming massflow according to:
      | mdot1 = mdot * fdiv
      | mdot2 = mdot * (1-fdiv)
      | fdiv is limited to the range [0..1]
      mask Help: web(fullfile(path_carnot('help'),'Flow_Diverter.html'),'-helpbrowser')
      mask Display: plot(0,-5,120,65,[20 45 20 20],[20 30 40 20],[45 70 70 45],[30 20 40 30],[45 35 55 45],[30 10 10 30])
  Flow_Mixer_basic : Subsystem  mask(Flow Mixer Basic){}
      mask help:
      | The flow mixer calculated the temperature and massflow of 2 entering flows.
      | The temperature is calculated in the block Mix_T_Mdot.
      | The flow diversion fdiv (feed back to the flow diverter) takes care that the pressure drop in the 2 branches is the same. The resulting pressure drop coefficients are calulated in the s-function mix_flow (uses solve_quadratic_equation in Carlib).
      mask Help: web(fullfile(path_carnot('help'),'Flow_Mixer_basic.html'),'-helpbrowser')
      mask Display: disp('Flow\nMixer')
  Icontrol_fdiv : Subsystem  AncestorBlock=carnot/Hydraulics/Flow_Mixer_Thermostatic/Icontrol_fdiv
  MinMax : MinMax  Inputs=2
  Mux : Mux  Inputs=2
  Mux1 : Mux  Inputs=2
  Mux2 : Mux  Inputs=3
  Mux3 : Mux  Inputs=3
  Product : Product  Inputs=3
  Scope : Scope  NumInputPorts=2
  Scope{1..8} (8 alike) : Scope
  Selector{,1..2,6} (4 alike) : Selector  InputPortWidth=2  IndexOptions=Index vector (dialog)  Indices=[1]  OutputSizes=1
  Selector{3..5,7} (4 alike) : Selector  InputPortWidth=2  IndexOptions=Index vector (dialog)  Indices=[2]  OutputSizes=1
  cp : Constant  Value=4185
  mdot1 : InitialCondition  Value=0.2
  mdot2 : InitialCondition  Value=28
  mdot_max : Constant  Value=mdot_d_w
  T_supply : Outport
  mdot_supply : Outport  Port=2
  mdot_2_sto : Outport  Port=3
  Q_supply : Outport  Port=4
  wires:
  Mux1/1 -> Flow_Mixer_basic/1(THB1), Selector4/1, Selector1/1
  Flow_Diverter/1(THB1) -> Selector5/1, Selector2/1, Flow_Mixer_basic/2(THB2), Scope4/1
  Mux2/1 -> Scope/1
  Mux3/1 -> Bias for display/1
  Bias for display/1 -> Scope/2
  Selector6/1 -> Icontrol_fdiv/1(Twarm)
  T_set/1 -> Icontrol_fdiv/2(Tset)
  T_return/1 -> Add/1, Mux/1
  Mux/1 -> Flow_Diverter/1(THB)
  Flow_Diverter/2(THB2) -> Selector7/1
  T_sto1/1 -> Mux1/1
  Selector7/1 -> Mux1/2, Scope3/1, mdot_2_sto/1
  Selector/1 -> Scope6/1, Add/2, T_supply/1, Mux2/1
  Selector1/1 -> Mux2/2
  Selector2/1 -> Mux2/3
  Selector4/1 -> Scope7/1, Mux3/2
  Selector5/1 -> Scope5/1, Mux3/3
  Selector3/1 -> Scope8/1, MinMax/1, Mux3/1
  mdot1/1 -> Mux/2
  MinMax/1 -> Product/3, Scope2/1, mdot_supply/1
  mdot_max/1 -> MinMax/2
  mdot_supply_in/1 -> mdot1/1
  Product/1 -> Q_supply/1
  Add/1 -> Product/1
  cp/1 -> Product/2
  Icontrol_fdiv/1(f_div) -> Scope1/1, Flow_Diverter/2(fdiv)
  Flow_Mixer_basic/1(THB) -> Selector3/1, Selector/1, mdot2/1
  mdot2/1 -> Selector6/1

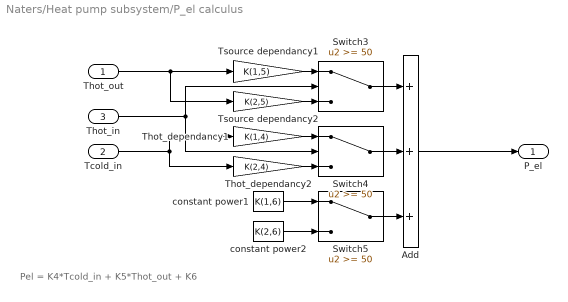
== system Naters/Heat pump subsystem/P_el calculus ==
  note: Pel = K4*Tcold_in + K5*Thot_out + K6
  Thot_out : Inport
  Tcold_in : Inport  Port=2
  Thot_in : Inport  Port=3
  Add : Sum  Inputs=+++
  Switch3 : Switch  Threshold=50
  Switch4 : Switch  Threshold=50
  Switch5 : Switch  Threshold=50
  Thot_dependancy1 : Gain  Gain=K(1,4)  SaturateOnIntegerOverflow=on  OutDataTypeStr=Inherit: Same as input  ParamDataTypeStr=Inherit: Same as input
  Thot_dependancy2 : Gain  Gain=K(2,4)  SaturateOnIntegerOverflow=on  OutDataTypeStr=Inherit: Same as input  ParamDataTypeStr=Inherit: Same as input
  Tsource dependancy1 : Gain  Gain=K(1,5)  SaturateOnIntegerOverflow=on  OutDataTypeStr=Inherit: Same as input  ParamDataTypeStr=Inherit: Same as input
  Tsource dependancy2 : Gain  Gain=K(2,5)  SaturateOnIntegerOverflow=on  OutDataTypeStr=Inherit: Same as input  ParamDataTypeStr=Inherit: Same as input
  constant power1 : Constant  Value=K(1,6)
  constant power2 : Constant  Value=K(2,6)
  P_el : Outport
  wires:
  Tcold_in/1 -> Thot_dependancy2/1, Thot_dependancy1/1
  Add/1 -> P_el/1
  Thot_out/1 -> Tsource dependancy2/1, Tsource dependancy1/1
  Switch3/1 -> Add/1
  Switch4/1 -> Add/2
  constant power1/1 -> Switch5/1
  Thot_in/1 -> Switch4/2, Switch3/2
  Tsource dependancy1/1 -> Switch3/1
  Tsource dependancy2/1 -> Switch3/3
  Thot_dependancy1/1 -> Switch4/1
  Thot_dependancy2/1 -> Switch4/3
  Switch5/1 -> Add/3
  constant power2/1 -> Switch5/3

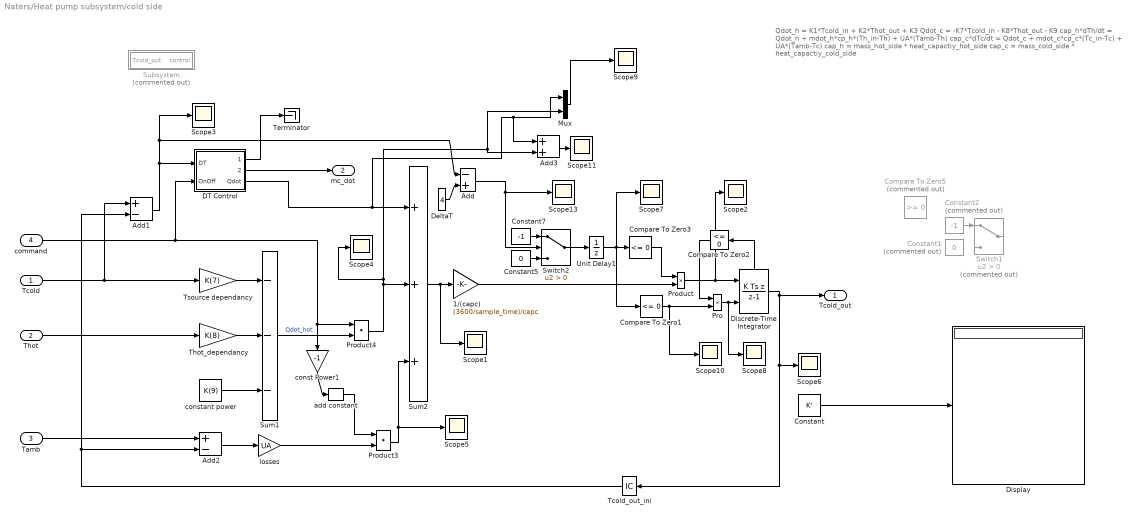
== system Naters/Heat pump subsystem/cold side ==
  note: Qdot_h = K1*Tcold_in + K2*Thot_out + K3
      |
      | Qdot_c = -K7*Tcold_in - K8*Thot_out - K9
      |
      | cap_h*dTh/dt = Qdot_h + mdot_h*cp_h*(Th_in-Th) + UA*(Tamb-Th)
      |
      | cap_c*dTc/dt = Qdot_c + mdot_c*cp_c*(Tc_in-Tc) + UA*(Tamb-Tc)
      |
      | cap_h = mass_hot_side * heat_capactiy_hot_side
      |
      | cap_c = mass_cold_side * heat_capactiy_cold_side
  Tcold : Inport
  Thot : Inport  Port=2
  Tamb : Inport  Port=3
  command : Inport  Port=4
  1/(capc) : Gain  Gain=(3600/sample_time)/capc
  Add : Sum  Inputs=-+
  Add1 : Sum  Inputs=+-
  Add2 : Sum  Inputs=+-
  Add3 : Sum
  Compare To Zero1 : simulink/Logic and Bit Operations/Compare To Zero  relop=<=  OutDataTypeStr=uint8
  Compare To Zero2 : simulink/Logic and Bit Operations/Compare To Zero  relop=<=  OutDataTypeStr=uint8
  Compare To Zero3 : simulink/Logic and Bit Operations/Compare To Zero  relop=<=  OutDataTypeStr=uint8
  Compare To Zero5 : simulink/Logic and Bit Operations/Compare To Zero  Commented=on  relop=>=  OutDataTypeStr=uint8
  Constant : Constant  Value=K'
  Constant1 : Constant  Commented=on  Value=0  SampleTime=-1
  Constant2 : Constant  Commented=on  Value=-1  SampleTime=-1
  Constant5 : Constant  Value=0  SampleTime=-1
  Constant7 : Constant  Value=-1  SampleTime=-1
  DT Control : Subsystem  mask{DTset=4, mcdotd=mcdot}
      mask prompts: DTset "Desired delta T on district heating network side"; mcdotd "design mass load on cold side [kg/s]"
  DeltaT : Constant  Value=4
  Discrete-Time Integrator : DiscreteIntegrator  IntegratorMethod=Integration: Backward Euler  ExternalReset=rising  InitialCondition=5.9  InitialConditionSetting=State (most efficient)  SampleTime=-1  ShowStatePort=on  ICPrevOutput=DiscIntNeverNeededParam  ICPrevScaledInput=DiscIntNeverNeededParam
  Display : Display
  Mux : Mux  Inputs=2
  Pro : Product
  Product : Product
  Product3 : DotProduct  InputSameDT=on  OutDataTypeStr=Inherit: Inherit via internal rule
  Product4 : DotProduct  InputSameDT=on  OutDataTypeStr=Inherit: Inherit via internal rule
  Scope{1..11,13} (12 alike) : Scope
  Subsystem : Subsystem  Commented=on
  Sum1 : Sum  Inputs=---  SaturateOnIntegerOverflow=on  InputSameDT=on  OutDataTypeStr=Inherit: Same as first input
  Sum2 : Sum  Inputs=+++  SaturateOnIntegerOverflow=on  InputSameDT=on  OutDataTypeStr=Inherit: Same as first input
  Switch1 : Switch  Commented=on  Criteria=u2 > Threshold
  Switch2 : Switch  Criteria=u2 > Threshold
  Tcold_out_ini : InitialCondition  Value=6.1
  Terminator : Terminator
  Thot_dependancy : Gain  Gain=K(8)  SaturateOnIntegerOverflow=on  OutDataTypeStr=Inherit: Same as input  ParamDataTypeStr=Inherit: Same as input
  Tsource dependancy : Gain  Gain=K(7)  SaturateOnIntegerOverflow=on  OutDataTypeStr=Inherit: Same as input  ParamDataTypeStr=Inherit: Same as input
  Unit Delay1 : UnitDelay  SampleTime=-1
  add constant : carnot/Basic/Thermal_Models/HeatPump_basic/model cold side/add constant  c=+1
  const Power1 : Gain  Gain=-1  SaturateOnIntegerOverflow=on  OutDataTypeStr=Inherit: Same as input  ParamDataTypeStr=Inherit: Same as input
  constant power : Constant  Value=K(9)
  losses : Gain  Gain=UA
  Tcold_out : Outport
  mc_dot : Outport  Port=2
  wires:
  Product4/1 -> Mux/2, Add3/2, Scope4/1, Sum2/2
  Sum2/1 -> 1/(capc)/1, Scope1/1
  const Power1/1 -> add constant/1
  add constant/1 -> Product3/1
  losses/1 -> Product3/2
  command/1 -> const Power1/1, Product4/1, DT Control/2(OnOff)
  Tamb/1 -> Add2/1
  Sum1/1 -> Product4/2  "Qdot_hot"
  constant power/1 -> Sum1/3
  Thot_dependancy/1 -> Sum1/2
  Tsource dependancy/1 -> Sum1/1
  Add2/1 -> losses/1
  Thot/1 -> Thot_dependancy/1
  Constant/1 -> Display/1
  Product3/1 -> Sum2/3, Scope5/1
  Discrete-Time Integrator/1 -> Tcold_out/1, Tcold_out_ini/1, Scope6/1
  DT Control/1(control) -> Terminator/1
  Mux/1 -> Scope9/1
  Tcold/1 -> Add1/1, Tsource dependancy/1
  Add3/1 -> Scope11/1
  DT Control/3(Qdot) -> Sum2/1, Add3/1, Mux/1
  1/(capc)/1 -> Product/2
  Constant7/1 -> Switch2/1
  Constant5/1 -> Switch2/3
  Switch2/1 -> Unit Delay1/1
  Product/1 -> Scope2/1, Discrete-Time Integrator/1
  DeltaT/1 -> Add/2
  Add1/1 -> Add/1, Scope3/1, DT Control/1(DT)
  Compare To Zero3/1 -> Product/1
  Tcold_out_ini/1 -> Add2/2, Add1/2
  DT Control/2(mcdot1) -> mc_dot/1
  Constant2/1 -> Switch1/1
  Add/1 -> Scope13/1, Switch2/2
  Compare To Zero1/1 -> Scope10/1, Pro/2
  Discrete-Time Integrator/State -> Compare To Zero2/1
  Compare To Zero2/1 -> Pro/1
  Pro/1 -> Scope8/1, Discrete-Time Integrator/2
  Unit Delay1/1 -> Compare To Zero1/1, Compare To Zero3/1, Scope7/1

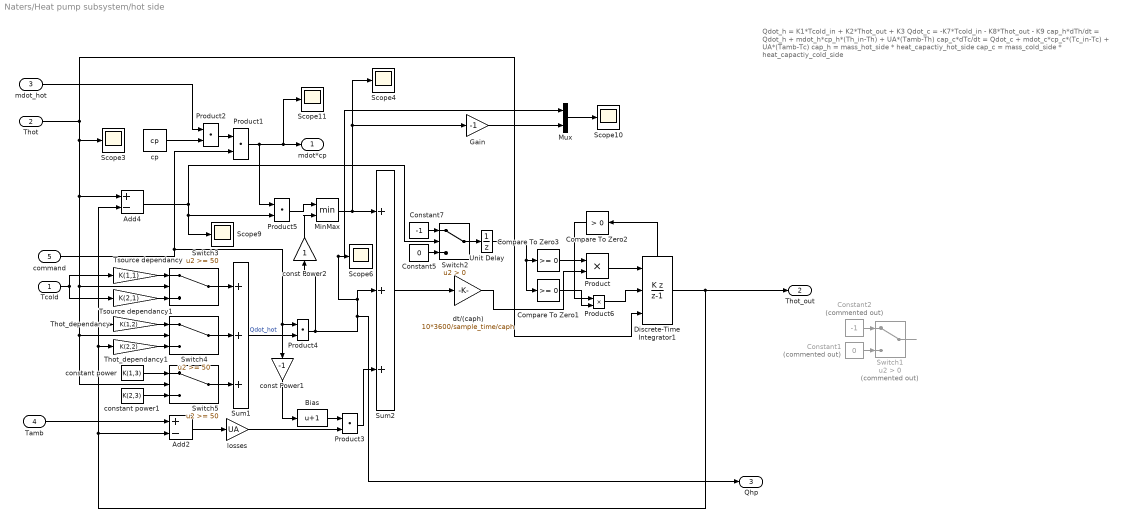
== system Naters/Heat pump subsystem/hot side ==
  note: Qdot_h = K1*Tcold_in + K2*Thot_out + K3
      |
      | Qdot_c = -K7*Tcold_in - K8*Thot_out - K9
      |
      | cap_h*dTh/dt = Qdot_h + mdot_h*cp_h*(Th_in-Th) + UA*(Tamb-Th)
      |
      | cap_c*dTc/dt = Qdot_c + mdot_c*cp_c*(Tc_in-Tc) + UA*(Tamb-Tc)
      |
      | cap_h = mass_hot_side * heat_capactiy_hot_side
      |
      | cap_c = mass_cold_side * heat_capactiy_cold_side
  Tcold : Inport
  Thot : Inport  Port=2
  mdot_hot : Inport  Port=3
  Tamb : Inport  Port=4
  command : Inport  Port=5
  Add2 : Sum  Inputs=+-
  Add4 : Sum  Inputs=+-
  Bias : Bias  Bias=1
  Compare To Zero1 : simulink/Logic and Bit Operations/Compare To Zero  relop=>=  OutDataTypeStr=uint8
  Compare To Zero2 : simulink/Logic and Bit Operations/Compare To Zero  relop=>  OutDataTypeStr=uint8
  Compare To Zero3 : simulink/Logic and Bit Operations/Compare To Zero  relop=>=  OutDataTypeStr=uint8
  Constant1 : Constant  Commented=on  Value=0  SampleTime=-1
  Constant2 : Constant  Commented=on  Value=-1  SampleTime=-1
  Constant5 : Constant  Value=0  SampleTime=-1
  Constant7 : Constant  Value=-1  SampleTime=-1
  Discrete-Time Integrator1 : DiscreteIntegrator  IntegratorMethod=Accumulation: Backward Euler  ExternalReset=falling  InitialConditionSource=external  InitialCondition=30  InitialConditionSetting=State (most efficient)  SampleTime=-1  UpperSaturationLimit=40  ShowStatePort=on  ICPrevOutput=DiscIntNeverNeededParam  ICPrevScaledInput=DiscIntNeverNeededParam
  Gain : Gain  Gain=-1
  MinMax : MinMax  Inputs=2
  Mux : Mux  Inputs=2
  Product : Product
  Product{1..5} (5 alike) : DotProduct  InputSameDT=on  OutDataTypeStr=Inherit: Inherit via internal rule
  Product6 : Product
  Scope{3..4,6,9..11} (6 alike) : Scope
  Sum1 : Sum  Inputs=+++  SaturateOnIntegerOverflow=on  InputSameDT=on  OutDataTypeStr=Inherit: Same as first input
  Sum2 : Sum  Inputs=+++  SaturateOnIntegerOverflow=on  InputSameDT=on  OutDataTypeStr=Inherit: Same as first input
  Switch1 : Switch  Commented=on  Criteria=u2 > Threshold
  Switch2 : Switch  Criteria=u2 > Threshold
  Switch3 : Switch  Threshold=50
  Switch4 : Switch  Threshold=50
  Switch5 : Switch  Threshold=50
  Thot_dependancy : Gain  Gain=K(1,2)  SaturateOnIntegerOverflow=on  OutDataTypeStr=Inherit: Same as input  ParamDataTypeStr=Inherit: Same as input
  Thot_dependancy1 : Gain  Gain=K(2,2)  SaturateOnIntegerOverflow=on  OutDataTypeStr=Inherit: Same as input  ParamDataTypeStr=Inherit: Same as input
  Tsource dependancy : Gain  Gain=K(1,1)  SaturateOnIntegerOverflow=on  OutDataTypeStr=Inherit: Same as input  ParamDataTypeStr=Inherit: Same as input
  Tsource dependancy1 : Gain  Gain=K(2,1)  SaturateOnIntegerOverflow=on  OutDataTypeStr=Inherit: Same as input  ParamDataTypeStr=Inherit: Same as input
  Unit Delay : UnitDelay  SampleTime=-1
  const Power1 : Gain  Gain=-1  SaturateOnIntegerOverflow=on  OutDataTypeStr=Inherit: Same as input  ParamDataTypeStr=Inherit: Same as input
  const Power2 : Gain  SaturateOnIntegerOverflow=on  OutDataTypeStr=Inherit: Same as input  ParamDataTypeStr=Inherit: Same as input
  constant power : Constant  Value=K(1,3)
  constant power1 : Constant  Value=K(2,3)
  cp : Constant  Value=cp
  dt/(caph) : Gain  Gain=10*3600/sample_time/caph
  losses : Gain  Gain=UA
  mdot*cp : Outport
  Thot_out : Outport  Port=2
  Qhp : Outport  Port=3
  wires:
  mdot_hot/1 -> Product2/1
  Add2/1 -> losses/1
  Switch3/1 -> Sum1/1
  Switch4/1 -> Sum1/2
  constant power/1 -> Switch5/1
  Sum1/1 -> Product4/2  "Qdot_hot"
  Tamb/1 -> Add2/1
  command/1 -> Product1/2, Product4/1, const Power1/1
  losses/1 -> Product3/2
  Bias/1 -> Product3/1
  const Power1/1 -> Bias/1
  Sum2/1 -> dt/(caph)/1
  Product3/1 -> Sum2/3
  Product4/1 -> const Power2/1, Qhp/1, Mux/1, Scope6/1, Sum2/2
  cp/1 -> Product2/2
  Product2/1 -> Product1/1
  Product1/1 -> Scope11/1, mdot*cp/1, Product5/1
  Mux/1 -> Scope10/1
  Gain/1 -> Mux/2
  MinMax/1 -> Gain/1, Scope4/1, Sum2/1
  Product5/1 -> MinMax/1
  const Power2/1 -> MinMax/2
  Add4/1 -> Scope9/1, Product5/2, Switch2/2
  Discrete-Time Integrator1/1 -> Thot_dependancy1/1, Add4/2, Thot_dependancy/1, Add2/2, Thot_out/1
  Constant7/1 -> Switch2/1
  Switch2/1 -> Unit Delay/1
  Constant5/1 -> Switch2/3
  Product/1 -> Discrete-Time Integrator1/1
  Compare To Zero3/1 -> Product/1
  Unit Delay/1 -> Compare To Zero1/1, Compare To Zero3/1
  dt/(caph)/1 -> Product/2
  ? -> Switch1/2
  Constant2/1 -> Switch1/1
  Switch1/1 -> ?
  Constant1/1 -> Switch1/3
  Compare To Zero1/1 -> Product6/2
  Thot/1 -> Discrete-Time Integrator1/3, Switch3/2, Switch4/2, Switch5/2, Add4/1, Scope3/1
  Product6/1 -> Discrete-Time Integrator1/2
  Discrete-Time Integrator1/State -> Compare To Zero2/1
  Compare To Zero2/1 -> Product6/1
  Tsource dependancy/1 -> Switch3/1
  Tcold/1 -> Tsource dependancy1/1, Tsource dependancy/1
  Tsource dependancy1/1 -> Switch3/3
  Thot_dependancy/1 -> Switch4/1
  Thot_dependancy1/1 -> Switch4/3
  Switch5/1 -> Sum1/3
  constant power1/1 -> Switch5/3

== system Naters/Space Heating Control/Trset ==
  Pulse Generator : DiscretePulseGenerator  PulseType=Time based  Amplitude=rep_seq_y  Period=period  PulseWidth=rep_seq_d*100/period  PhaseDelay=rep_seq_t
  Sum of Elements : Sum  Inputs=+
  Trset : Outport
  wires:
  Pulse Generator/1 -> Sum of Elements/1
  Sum of Elements/1 -> Trset/1

== system Naters/Space Heating Control/controller ==
  Tamb : Inport
  Trset : Inport  Port=2
  Fcn : Fcn  Expr=Q_LOC*3.6*(u(2)-u(1))/(u(2)-Tambd)
  Fcn1 : Fcn  Expr=Tset+(u(1)/(Q_LOC*3.6))^(1/n_rad)*(0.5*(Td_in + Td_out) - u(2))+u(1)/(2*Q_LOC*3.6)*(Td_in-Td_out)
  Mux1 : Mux  Inputs=2
  Mux2 : Mux  Inputs=2
  Saturation1 : Saturate  UpperLimit=inf  LowerLimit=0
  Scope{1..4,6} (5 alike) : Scope
  Tset : Outport
  wires:
  Tamb/1 -> Mux2/1
  Fcn/1 -> Scope2/1, Saturation1/1
  Fcn1/1 -> Tset/1
  Saturation1/1 -> Scope3/1, Mux1/1
  Mux2/1 -> Scope1/1, Fcn/1
  Trset/1 -> Scope4/1, Mux1/2, Mux2/2
  Mux1/1 -> Scope6/1, Fcn1/1

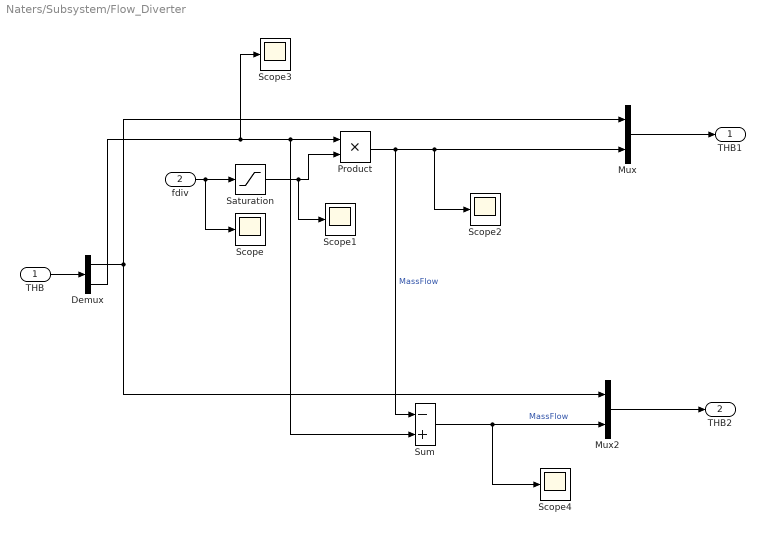
== system Naters/Subsystem/Flow_Diverter ==
  THB : Inport
  fdiv : Inport  Port=2
  Demux : Demux  Outputs=2
  Mux : Mux  Inputs=2
  Mux2 : Mux  Inputs=2
  Product : Product
  Saturation : Saturate  UpperLimit=1  LowerLimit=0
  Scope{,1..4} (5 alike) : Scope
  Sum : Sum  Inputs=-+  SaturateOnIntegerOverflow=on  InputSameDT=on  OutDataTypeStr=Inherit: Same as first input
  THB1 : Outport
  THB2 : Outport  Port=2
  wires:
  Saturation/1 -> Product/2, Scope1/1
  Sum/1 -> Scope4/1, Mux2/2  "MassFlow"
  Demux/2 -> Scope3/1, Product/1, Sum/2
  fdiv/1 -> Scope/1, Saturation/1
  Product/1 -> Sum/1, Scope2/1, Mux/2  "MassFlow"
  Mux/1 -> THB1/1
  Mux2/1 -> THB2/1
  THB/1 -> Demux/1
  Demux/1 -> Mux/1, Mux2/1

== system Naters/Subsystem/Flow_Mixer_basic ==
  THB1 : Inport
  THB2 : Inport  Port=2
  Mix_T_Mdot : Subsystem  mask(mix_temperature){mixcalc=Tmix = (mdot1*T1 + mdot2*T2)/(mdot1+mdot2)}
      mask prompts: mixcalc "Calculation of mixture :"
      mask help:
      | Calculate the temperature of the mixture of two flows. Uses enthalpy balance for humid air. Liquids may be mixed by the (faster and approximate) equation:
      | Tmix = (mdot1*T1 + mdot2*T2)/(mdot1+mdot2)
      mask Help: web(fullfile(path_carnot('help'),'Mix_T_Mdot.html'),'-helpbrowser')
      mask TypeOptions mixcalc: Tmix = (mdot1*T1 + mdot2*T2)/(mdot1+mdot2) | Enthalpy balance
  Mux : Mux  Inputs=2
  THB : Outport
  wires:
  THB1/1 -> Mix_T_Mdot/1(THB1)
  THB2/1 -> Mix_T_Mdot/2(THB2)
  Mix_T_Mdot/1(T) -> Mux/1  "T"
  Mix_T_Mdot/2(mdot) -> Mux/2
  Mux/1 -> THB/1

== system Naters/Subsystem/Icontrol_fdiv ==
  Twarm : Inport
  Tset : Inport  Port=2
  (Discrete-Time Integrator)1 : DiscreteIntegrator  IntegratorMethod=Integration: Backward Euler  gainval=1  InitialCondition=1  InitialConditionSetting=State (most efficient)  SampleTime=-1  LimitOutput=on  UpperSaturationLimit=1  LowerSaturationLimit=0  ICPrevOutput=DiscIntNeverNeededParam  ICPrevScaledInput=DiscIntNeverNeededParam
  Gain : Gain  Gain=20*(sample_time-5)/sample_time  SaturateOnIntegerOverflow=on  OutDataTypeStr=Inherit: Same as input  ParamDataTypeStr=Inherit: Same as input
  diff_T : Sum  Inputs=+-  SaturateOnIntegerOverflow=on  InputSameDT=on  OutDataTypeStr=Inherit: Same as first input
  f_div : Outport
  wires:
  diff_T/1 -> Gain/1
  Twarm/1 -> diff_T/1
  Tset/1 -> diff_T/2
  (Discrete-Time Integrator)1/1 -> f_div/1
  Gain/1 -> (Discrete-Time Integrator)1/1
